simulink model "gtm_design"  (R2019b)
settings: Solver=ode3  StartTime=0.0  StopTime=Inf  FixedStep=Timestep  MaxStep=.1  RelTol=1e-5
InitFcn:
  | if ~exist('MAG3TempComp','var')
  |     appendmws(Cal_params_T2)
  | end
StopFcn:
  | MWSout=grabmws(bdroot);
  | MWSout.lastrun=datestr(now);
undefined symbols (not defined in the file): Aero, aftfuel, aftfuel_pos, b, bias, Cbar, cg_pos0, cg_shift_gear, DamageCase, DamageModels, DamageOnsetTime, engl_ang, engl_pos, engr_ang, engr_pos, fwdfuel, fwdfuel_pos, Inertia0, Inertia_shift_gear, ref_cg, runway_alt, S, StatesInp, symmetric_aero_on, Timestep, w0, WindDir, WindSpd
libraries: simulink_need_slupdate x28, Servo_Model_lib x18, simulink x4, Polyval_lib x3, GTM_aerolib x2, Cross_Product_3D_lib x2, Euler_to_DCM_lib x1, Vb_Converter_lib x1, eomlib x1, sensors_T2_design_lib x1, Doublet_Generator_lib x1, NamedStore_lib x1
(part 1 of 2)
settings Model: ExtModeAutoUpdateStatusClock=off  OrderedModelArguments=off  Creator=cox  LastModifiedBy=suvo
settings DataIOCC: LimitDataPoints=on  MaxDataPoints=50000  SaveFormat=Structure  SignalLoggingSaveFormat=ModelDataLogs  SaveOutput=off  SignalLogging=off  ReturnWorkspaceOutputs=off
settings OptimizationCC: BooleanDataType=off  ExpressionDepthLimit=2147483647  InitFltsAndDblsToZero=on  LifeSpan=inf
settings DebuggingCC: SaveWithParameterizedLinksMsg=none  UnderspecifiedInitializationDetection=Classic  MergeDetectMultiDrivingBlocksExec=none  SignalResolutionControl=TryResolveAllWithWarning  InheritedTsInSrcMsg=none  MultiTaskDSMMsg=warning  MultiTaskCondExecSysMsg=none  FcnCallInpInsideContextMsg=warning  StateNameClashWarn=warning  InitInArrayFormatMsg=none  SFUnexpectedBacktrackingDiag=warning  SFNoUnconditionalDefaultTransitionDiag=warning  SFExecutionAtInitializationDiag=none  ArithmeticOperatorsInVariantConditions=warning
settings HardwareCC: ProdBitPerPointer=32  ProdBitPerSizeT=32  ProdBitPerPtrDiffT=32  ProdLargestAtomicFloat=None  ProdIntDivRoundTo=Undefined  ProdEndianess=Unspecified  ProdWordSize=32  ProdHWDeviceType=32-bit Generic  TargetHWDeviceType=32-bit Generic
settings ModelReferenceCC: PropagateSignalLabelsOutOfModel=off
settings SFSimCC: SimUseLocalCustomCode=off  CustomCodeUndefinedFunction=UseInterfaceOnly
settings RTWCC: RTWUseLocalCustomCode=off
settings CodeAppCC: StateflowObjectComments=on
settings GRTTargetCC: TargetFcnLib=ansi_tfl_tmw.mat  TargetLangStandard=C89/C90 (ANSI)  CombineOutputUpdateFcns=off  GRTInterface=on
settings ConfigComp: CovMetricSettings=dw  CovHtmlReporting=on  CovSaveCumulativeToWorkspaceVar=on  CovSaveSingleToWorkspaceVar=on  CovExternalEMLEnable=off

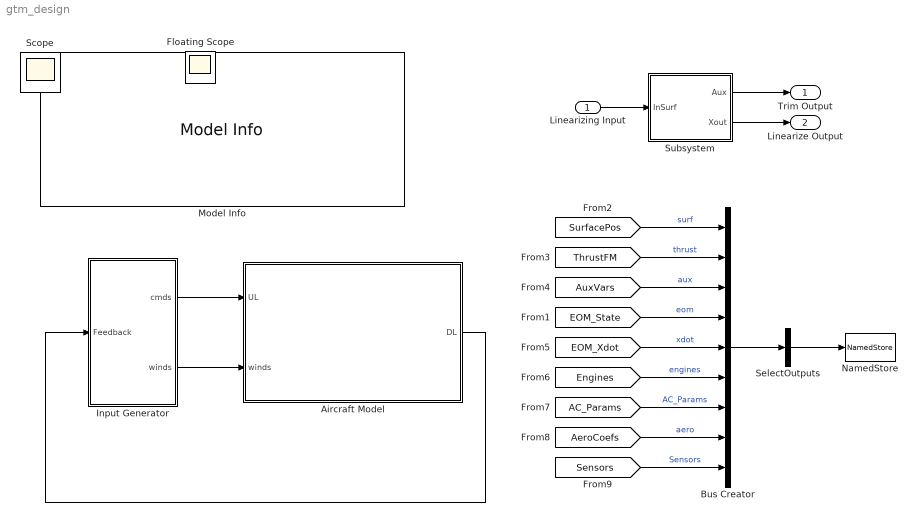
== system gtm_design ==
  Linearizing Input : Inport
  Aircraft Model : Subsystem  Tag=From trunk/GTMsim/gtm_model.mdl revision 162  BlockChoice=GTM_T2
      mask Display: image(imread('GTMtiny.png'))
  Bus Creator : BusCreator  Inputs=9
  Input Generator : Subsystem
  Model Info : simulink/Model-Wide Utilities/Model Info  Frame=on  DisplayStringWithTags=|  HorizontalTextAlignment=Center  LeftAlignmentValue=0.5
      | GTM Design-Simulation Model
      | Subversion Info: %<ModelVersion>
      | Last modified by %<LastModifiedBy> on %<LastModificationDate>
      | 
      | Copyright 2009
      | United States Government as represented by the 
      | Administrator of the National and Aeronautics and Space Administration.
      | 
      | No copyright is claimed in the United States under Title 17, U.S. Code.
      | All Other Rights Reserved.
  NamedStore : NamedStore_lib/NamedStore  Npts=inf  VarName=sout  expand=off
  SelectOutputs : BusSelector  OutputSignals=aux.eas,aux.alpha,aux.beta,aux.gamma  OutputAsBus=on
  Subsystem : Subsystem
  Trim Output : Outport  VectorParamsAs1DForOutWhenUnconnected=off
  Linearize Output : Outport  Port=2  VectorParamsAs1DForOutWhenUnconnected=off
  Floating Scope : Scope
  Scope : Scope
  wires:
  SelectOutputs/1 -> NamedStore/1
  [SurfacePos] -> Bus Creator/1  "surf"
  Linearizing Input/1 -> Subsystem/1(InSurf)
  Subsystem/1(Aux) -> Trim Output/1
  [EOM_State] -> Bus Creator/4  "eom"
  [AuxVars] -> Bus Creator/3  "aux"
  [ThrustFM] -> Bus Creator/2  "thrust"
  Subsystem/2(Xout) -> Linearize Output/1
  [EOM_Xdot] -> Bus Creator/5  "xdot"
  [Engines] -> Bus Creator/6  "engines"
  [AC_Params] -> Bus Creator/7  "AC_Params"
  Bus Creator/1 -> SelectOutputs/1
  Input Generator/1(cmds) -> Aircraft Model/1(UL)
  Input Generator/2(winds) -> Aircraft Model/2(winds)
  Aircraft Model/1(DL) -> Input Generator/1(Feedback)
  [AeroCoefs] -> Bus Creator/8  "aero"
  [Sensors] -> Bus Creator/9  "Sensors"

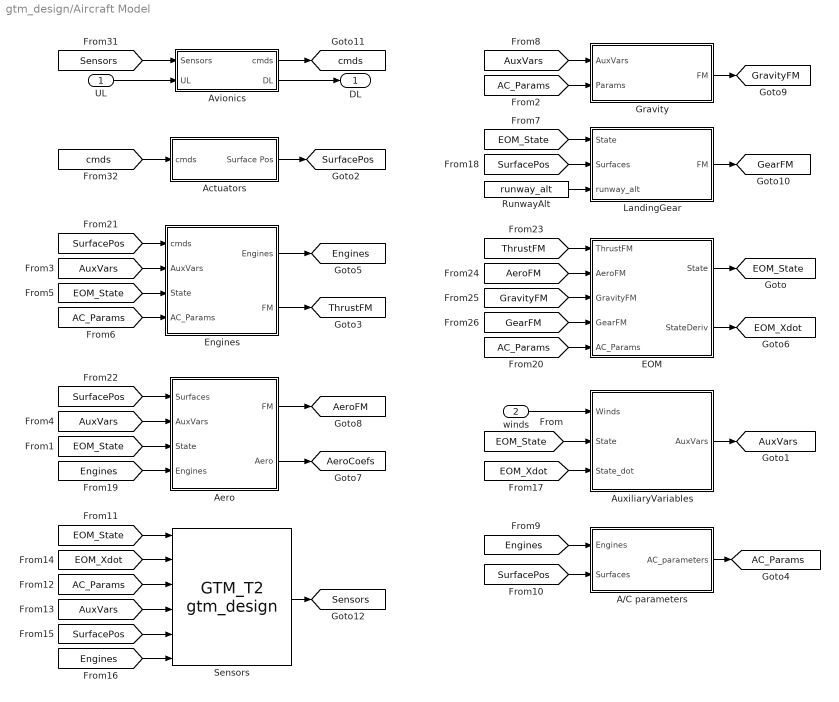
== system gtm_design/Aircraft Model ==
  UL : Inport
  winds : Inport  Port=2  PortDimensions=3
  A/C parameters : Subsystem
  Actuators : Subsystem
  Aero : Subsystem
  AuxiliaryVariables : Subsystem
  Avionics : Subsystem
  EOM : Subsystem
  Engines : Subsystem
  Gravity : Subsystem
  LandingGear : Subsystem  mask(LandingGear){GEAR_SPRING=25*12, zeta=0.4, NoseWheelRate=0.15}
      mask prompts: GEAR_SPRING "Gear Spring Constant (lbs/ft)"; zeta "Damping Factor"; NoseWheelRate "Nose Wheel Sensitivity"
      mask help: Landing Gear Model
  RunwayAlt : Constant  Value=runway_alt
  Sensors : sensors_T2_design_lib/GTM_T2 gtm_design  SystemSampleTime=-1  Latency=0  AutoFrameSizeCalculation=off
  DL : Outport  VectorParamsAs1DForOutWhenUnconnected=off
  tag scope: AC_Params=global, AeroCoefs=global, AeroFM=global, AuxVars=global, EOM_State=global, EOM_Xdot=global, Engines=global, GearFM=global, GravityFM=global, Sensors=global, SurfacePos=global, ThrustFM=global, cmds=global
  wires:
  Sensors/1 -> [Sensors]
  [cmds] -> Actuators/1(cmds)
  [Sensors] -> Avionics/1(Sensors)
  Avionics/1(cmds) -> [cmds]
  winds/1 -> AuxiliaryVariables/1(Winds)
  Actuators/1(Surface Pos) -> [SurfacePos]
  LandingGear/1(FM) -> [GearFM]
  [SurfacePos] -> LandingGear/2(Surfaces)
  [EOM_State] -> LandingGear/1(State)
  [EOM_State] -> Aero/3(State)
  AuxiliaryVariables/1(AuxVars) -> [AuxVars]
  [AuxVars] -> Aero/2(AuxVars)
  Aero/1(FM) -> [AeroFM]
  Engines/2(FM) -> [ThrustFM]
  EOM/1(State) -> [EOM_State]
  [AC_Params] -> Gravity/2(Params)
  [AuxVars] -> Gravity/1(AuxVars)
  [EOM_State] -> Engines/3(State)
  [AuxVars] -> Engines/2(AuxVars)
  [AC_Params] -> Engines/4(AC_Params)
  A/C parameters/1(AC_parameters) -> [AC_Params]
  [Engines] -> A/C parameters/1(Engines)
  [SurfacePos] -> A/C parameters/2(Surfaces)
  Engines/1(Engines) -> [Engines]
  [EOM_Xdot] -> AuxiliaryVariables/3(State_dot)
  [Engines] -> Aero/4(Engines)
  EOM/2(StateDeriv) -> [EOM_Xdot]
  [SurfacePos] -> Engines/1(cmds)
  RunwayAlt/1 -> LandingGear/3(runway_alt)
  [SurfacePos] -> Aero/1(Surfaces)
  Aero/2(Aero) -> [AeroCoefs]
  [EOM_State] -> AuxiliaryVariables/2(State)
  [ThrustFM] -> EOM/1(ThrustFM)
  [AeroFM] -> EOM/2(AeroFM)
  [GravityFM] -> EOM/3(GravityFM)
  [GearFM] -> EOM/4(GearFM)
  [AC_Params] -> EOM/5(AC_Params)
  [EOM_State] -> Sensors/1
  [AC_Params] -> Sensors/3
  [SurfacePos] -> Sensors/5
  [Engines] -> Sensors/6
  [EOM_Xdot] -> Sensors/2
  [AuxVars] -> Sensors/4
  Gravity/1(FM) -> [GravityFM]
  Avionics/2(DL) -> DL/1
  UL/1 -> Avionics/2(UL)

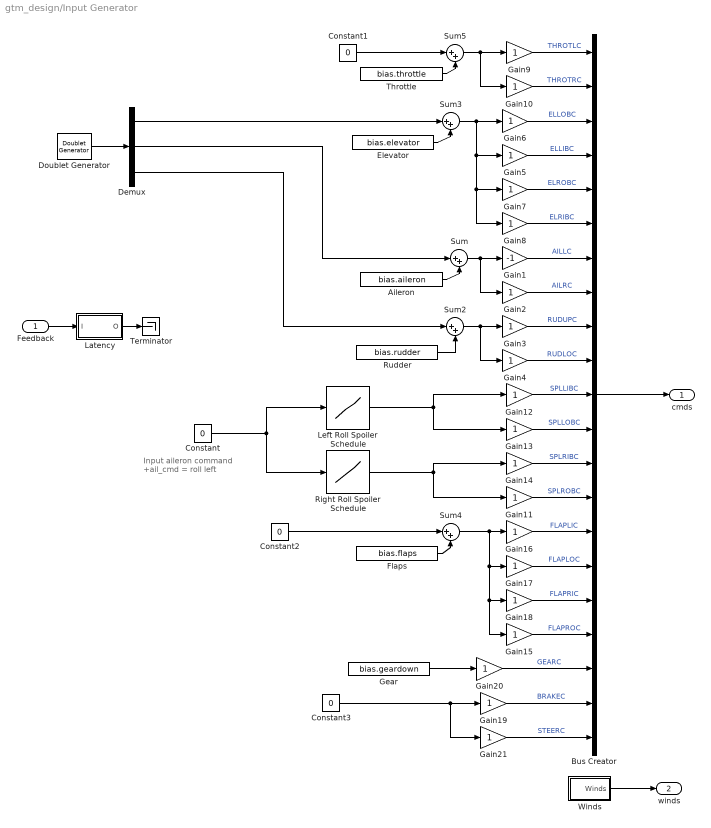
== system gtm_design/Input Generator ==
  note: Input aileron command
      | +ail_cmd = roll left
  Feedback : Inport
  Aileron : Constant  Value=bias.aileron
  Bus Creator : BusCreator  Inputs=21
  Constant{,1..3} (4 alike) : Constant  Value=0
  Demux : Demux  Outputs=3
  Doublet Generator : Doublet_Generator_lib/Doublet Generator  timeon=[2 12 7]  pulsewidth=[0.5 0.5 0.5]  amplitude=[0 0 0]
  Elevator : Constant  Value=bias.elevator
  Flaps : Constant  Value=bias.flaps
  Gain1 : Gain  Gain=-1  SaturateOnIntegerOverflow=on  OutDataTypeStr=Inherit: Same as input  ParamDataTypeStr=Inherit: Same as input
  Gain{2..21} (20 alike) : Gain  SaturateOnIntegerOverflow=on  OutDataTypeStr=Inherit: Same as input  ParamDataTypeStr=Inherit: Same as input
  Gear : Constant  Value=bias.geardown
  Latency : Subsystem
  Left Roll Spoiler Schedule : Lookup  InputValues="[-20\t-11.76\t-2.36\t0\t2.36\t11.76\t20\t]"  Table=[0 0 0 0 0 9 45]  LookUpMeth=Interpolation-Use End Values
  Right Roll Spoiler Schedule : Lookup  InputValues="[-20\t-11.76\t-2.36\t0\t2.36\t11.76\t20\t]"  Table=[45 9 0 0 0 0 0]  LookUpMeth=Interpolation-Use End Values
  Rudder : Constant  Value=bias.rudder
  Sum{,2..5} (5 alike) : Sum  Inputs=|++
  Terminator : Terminator
  Throttle : Constant  Value=bias.throttle
  Winds : Subsystem
  cmds : Outport  VectorParamsAs1DForOutWhenUnconnected=off
  winds : Outport  Port=2  VectorParamsAs1DForOutWhenUnconnected=off
  wires:
  Latency/1(O) -> Terminator/1
  Winds/1(Winds) -> winds/1
  Constant/1 -> Right Roll Spoiler Schedule/1, Left Roll Spoiler Schedule/1
  Right Roll Spoiler Schedule/1 -> Gain11/1, Gain14/1
  Left Roll Spoiler Schedule/1 -> Gain13/1, Gain12/1
  Gain12/1 -> Bus Creator/11  "SPLLIBC"
  Gain13/1 -> Bus Creator/12  "SPLLOBC"
  Gain14/1 -> Bus Creator/13  "SPLRIBC"
  Gain11/1 -> Bus Creator/14  "SPLROBC"
  Gain16/1 -> Bus Creator/15  "FLAPLIC"
  Gain17/1 -> Bus Creator/16  "FLAPLOC"
  Gain18/1 -> Bus Creator/17  "FLAPRIC"
  Gain15/1 -> Bus Creator/18  "FLAPROC"
  Gain9/1 -> Bus Creator/1  "THROTLC"
  Gain10/1 -> Bus Creator/2  "THROTRC"
  Gain5/1 -> Bus Creator/4  "ELLIBC"
  Gain6/1 -> Bus Creator/3  "ELLOBC"
  Gain7/1 -> Bus Creator/5  "ELROBC"
  Gain8/1 -> Bus Creator/6  "ELRIBC"
  Gain1/1 -> Bus Creator/7  "AILLC"
  Gain2/1 -> Bus Creator/8  "AILRC"
  Gain3/1 -> Bus Creator/9  "RUDUPC"
  Gain4/1 -> Bus Creator/10  "RUDLOC"
  Throttle/1 -> Sum5/2
  Constant1/1 -> Sum5/1
  Sum5/1 -> Gain10/1, Gain9/1
  Sum3/1 -> Gain6/1, Gain5/1, Gain7/1, Gain8/1
  Aileron/1 -> Sum/2
  Elevator/1 -> Sum3/2
  Sum/1 -> Gain1/1, Gain2/1
  Sum2/1 -> Gain3/1, Gain4/1
  Rudder/1 -> Sum2/2
  Flaps/1 -> Sum4/2
  Constant2/1 -> Sum4/1
  Sum4/1 -> Gain16/1, Gain17/1, Gain18/1, Gain15/1
  Doublet Generator/1 -> Demux/1
  Demux/2 -> Sum/1
  Demux/3 -> Sum2/1
  Gain19/1 -> Bus Creator/20  "BRAKEC"
  Gear/1 -> Gain20/1
  Constant3/1 -> Gain19/1, Gain21/1
  Demux/1 -> Sum3/1
  Bus Creator/1 -> cmds/1
  Feedback/1 -> Latency/1(I)
  Gain20/1 -> Bus Creator/19  "GEARC"
  Gain21/1 -> Bus Creator/21  "STEERC"

== system gtm_design/Subsystem ==
  InSurf : Inport
  Bus Selector : BusSelector  OutputSignals=eas,tas,alpha,beta,gamma,gndtrack  OutputAsBus=on
  Bus to Vector : BusToVector
  Bus to Vector1 : BusToVector
  DocBlock : simulink/Model-Wide Utilities/DocBlock  DocumentType=Text
      content=|
      | Inputs and Outputs selected here have a specific ordering.
      |
      |
      |
      | Do not change this without also changing output channel ordering in associated linmodel.m and
      | trimgtm.m functions
  Aux : Outport  VectorParamsAs1DForOutWhenUnconnected=off
  Xout : Outport  Port=2  VectorParamsAs1DForOutWhenUnconnected=off
  tag scope: SurfaceDeltas=global
  wires:
  [AuxVars] -> Bus Selector/1  "aux"
  [EOM_State] -> Bus to Vector1/1  "eom"
  Bus Selector/1 -> Bus to Vector/1
  InSurf/1 -> [SurfaceDeltas]
  Bus to Vector/1 -> Aux/1
  Bus to Vector1/1 -> Xout/1

== system gtm_design/Aircraft Model/A//C parameters ==
  Engines : Inport
  Surfaces : Inport  Port=2
  B : Constant  Value=b
  Bus Creator4 : BusCreator  Inputs=15
  Bus Selector : BusSelector  OutputSignals=fuel_used
  Bus Selector1 : BusSelector  OutputSignals=GEAR
  Cbar : Constant  Value=Cbar
  Demux : Demux  Outputs=6
  Inertia/Mass/CG Shift : Subsystem  mask{DamageModels=DamageModels}
      mask prompts: DamageModels "Array of Damage Cases"
      mask init:
      | Ncases=length(DamageModels);
      | dCGDamage=zeros(Ncases+1,3);   
      | dMassDamage=zeros(Ncases+1,1);
      | dInertiaDamage=zeros(Ncases+1,6);
      | for i=1:Ncases,
      |   if isfield(DamageModels{i},'Mass'),
      |      dInertiaDamage(i+1,:)=DamageModels{i}.Mass.dIxxIyyIzzIxzIyzIxy;
      |      dCGDamage(i+1,:)=DamageModels{i}.Mass.dCG;
      |      dMassDamage(i+1)=DamageModels{i}.Mass.dWeight;
      |   end
      | end
  S : Constant  Value=S
  TriggerDamage : Subsystem
  ixxb5 : Constant  Value=engr_pos
  ixxb6 : Constant  Value=engl_pos
  xCG1 : Constant  Value=ref_cg
  AC_parameters : Outport  VectorParamsAs1DForOutWhenUnconnected=off
  wires:
  Bus Selector/1 -> Inertia/Mass/CG Shift/2(fuel_used)  "<fuel_used>"
  Bus Selector1/1 -> Inertia/Mass/CG Shift/1(gear)  "<GEAR>"
  [DamageCase] -> Inertia/Mass/CG Shift/3(DamageCase)
  [DamageCase] -> Bus Creator4/13  "DamageCase"
  Inertia/Mass/CG Shift/3(CG) -> Bus Creator4/12  "CG"
  Inertia/Mass/CG Shift/2(mass) -> Bus Creator4/11  "mass"
  Demux/6 -> Bus Creator4/10  "Ixy"
  Demux/5 -> Bus Creator4/9  "Iyz"
  Demux/4 -> Bus Creator4/8  "Ixz"
  Demux/3 -> Bus Creator4/7  "Izz"
  Demux/2 -> Bus Creator4/6  "Iyy"
  Demux/1 -> Bus Creator4/5  "Ixx"
  ixxb6/1 -> Bus Creator4/15  "LfEng"
  ixxb5/1 -> Bus Creator4/14  "RtEng"
  xCG1/1 -> Bus Creator4/4  "CP"
  B/1 -> Bus Creator4/3  "B"
  Cbar/1 -> Bus Creator4/2  "Cbar"
  S/1 -> Bus Creator4/1  "S"
  TriggerDamage/1(damagecase) -> [DamageCase]
  Inertia/Mass/CG Shift/1(Inertia) -> Demux/1
  Surfaces/1 -> Bus Selector1/1
  Engines/1 -> Bus Selector/1
  Bus Creator4/1 -> AC_parameters/1

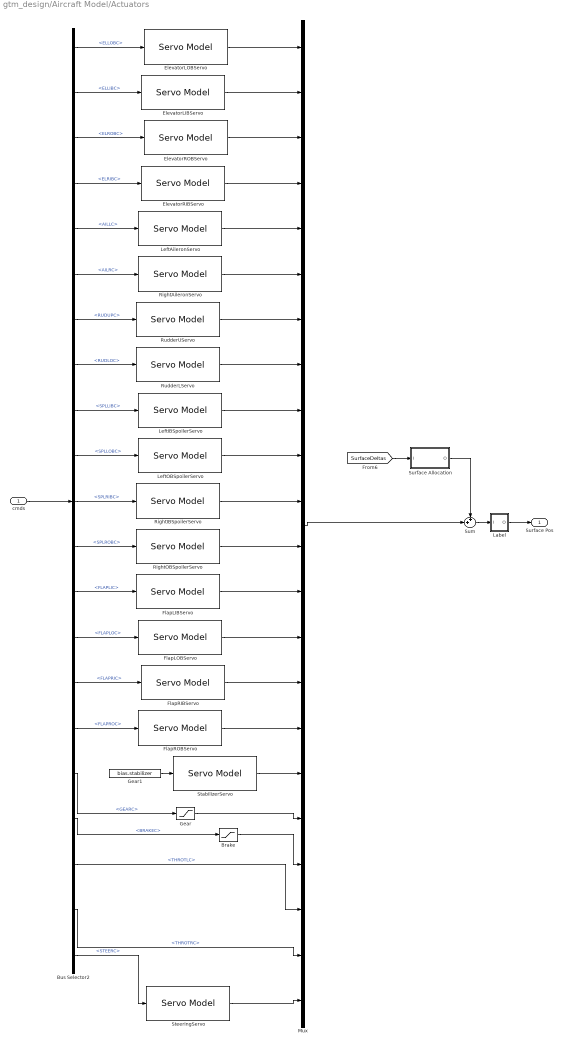
== system gtm_design/Aircraft Model/Actuators ==
  cmds : Inport
  Brake : Saturate  UpperLimit=1.0  LowerLimit=0.0
  Bus Selector2 : BusSelector  OutputSignals=ELLOBC,ELLIBC,ELROBC,ELRIBC,AILLC,AILRC,RUDUPC,RUDLOC,SPLLIBC,SPLLOBC,SPLRIBC,SPLROBC,FLAPLIC,FLAPLOC,FLAPRIC,FLAPROC,GEARC,BRAKEC,THROTLC,THROTRC,STEERC
  ElevatorLIBServo : Servo_Model_lib/Servo Model  freq=10  RL=300  POS_hi=20  POS_lo=-30  Bias=0
  ElevatorLOBServo : Servo_Model_lib/Servo Model  freq=10  RL=300  POS_hi=20  POS_lo=-30  Bias=0
  ElevatorRIBServo : Servo_Model_lib/Servo Model  freq=10  RL=300  POS_hi=20  POS_lo=-30  Bias=0
  ElevatorROBServo : Servo_Model_lib/Servo Model  freq=10  RL=300  POS_hi=20  POS_lo=-30  Bias=0
  FlapLIBServo : Servo_Model_lib/Servo Model  freq=10  RL=300  POS_hi=30  POS_lo=0  Bias=0
  FlapLOBServo : Servo_Model_lib/Servo Model  freq=10  RL=300  POS_hi=30  POS_lo=0  Bias=0
  FlapRIBServo : Servo_Model_lib/Servo Model  freq=10  RL=300  POS_hi=30  POS_lo=0  Bias=0
  FlapROBServo : Servo_Model_lib/Servo Model  freq=10  RL=300  POS_hi=30  POS_lo=0  Bias=0
  Gear : Saturate  UpperLimit=1.0  LowerLimit=0.0
  Gear1 : Constant  Value=bias.stabilizer
  Label : Subsystem
  LeftAileronServo : Servo_Model_lib/Servo Model  freq=10  RL=300  POS_hi=20.0  POS_lo=-20  Bias=0
  LeftIBSpoilerServo : Servo_Model_lib/Servo Model  freq=10  RL=300  POS_hi=15  POS_lo=0  Bias=0
  LeftOBSpoilerServo : Servo_Model_lib/Servo Model  freq=10  RL=300  POS_hi=45  POS_lo=0  Bias=0
  Mux : Mux  Inputs=22
  RightAileronServo : Servo_Model_lib/Servo Model  freq=10  RL=300  POS_hi=20.0  POS_lo=-20  Bias=0
  RightIBSpoilerServo : Servo_Model_lib/Servo Model  freq=10  RL=300  POS_hi=15  POS_lo=0  Bias=0
  RightOBSpoilerServo : Servo_Model_lib/Servo Model  freq=10  RL=300  POS_hi=45  POS_lo=0  Bias=0
  RudderLServo : Servo_Model_lib/Servo Model  freq=8.43  RL=300  POS_hi=30  POS_lo=-30.0  Bias=0
  RudderUServo : Servo_Model_lib/Servo Model  freq=8.43  RL=300  POS_hi=30  POS_lo=-30.0  Bias=0
  StabilizerServo : Servo_Model_lib/Servo Model  freq=10  RL=300  POS_hi=4  POS_lo=-12  Bias=0
  SteeringServo : Servo_Model_lib/Servo Model  freq=10  RL=300  POS_hi=30  POS_lo=0  Bias=0
  Sum : Sum  Inputs=++|
  Surface Allocation : Subsystem
  Surface Pos : Outport  VectorParamsAs1DForOutWhenUnconnected=off
  wires:
  SteeringServo/1 -> Mux/22
  Bus Selector2/21 -> SteeringServo/1  "<STEERC>"
  Bus Selector2/20 -> Mux/21  "<THROTRC>"
  Bus Selector2/19 -> Mux/20  "<THROTLC>"
  Gear1/1 -> StabilizerServo/1
  Surface Allocation/1(O) -> Sum/1
  cmds/1 -> Bus Selector2/1
  Brake/1 -> Mux/19
  Gear/1 -> Mux/18
  StabilizerServo/1 -> Mux/17
  FlapROBServo/1 -> Mux/16
  FlapRIBServo/1 -> Mux/15
  FlapLOBServo/1 -> Mux/14
  FlapLIBServo/1 -> Mux/13
  RightOBSpoilerServo/1 -> Mux/12
  RightIBSpoilerServo/1 -> Mux/11
  LeftOBSpoilerServo/1 -> Mux/10
  LeftIBSpoilerServo/1 -> Mux/9
  RudderLServo/1 -> Mux/8
  Bus Selector2/12 -> RightOBSpoilerServo/1  "<SPLROBC>"
  Bus Selector2/11 -> RightIBSpoilerServo/1  "<SPLRIBC>"
  Bus Selector2/10 -> LeftOBSpoilerServo/1  "<SPLLOBC>"
  Bus Selector2/9 -> LeftIBSpoilerServo/1  "<SPLLIBC>"
  Bus Selector2/8 -> RudderLServo/1  "<RUDLOC>"
  Bus Selector2/7 -> RudderUServo/1  "<RUDUPC>"
  RudderUServo/1 -> Mux/7
  RightAileronServo/1 -> Mux/6
  Bus Selector2/6 -> RightAileronServo/1  "<AILRC>"
  LeftAileronServo/1 -> Mux/5
  Bus Selector2/5 -> LeftAileronServo/1  "<AILLC>"
  ElevatorRIBServo/1 -> Mux/4
  Bus Selector2/4 -> ElevatorRIBServo/1  "<ELRIBC>"
  ElevatorROBServo/1 -> Mux/3
  Bus Selector2/3 -> ElevatorROBServo/1  "<ELROBC>"
  ElevatorLIBServo/1 -> Mux/2
  ElevatorLOBServo/1 -> Mux/1
  Bus Selector2/2 -> ElevatorLIBServo/1  "<ELLIBC>"
  Bus Selector2/1 -> ElevatorLOBServo/1  "<ELLOBC>"
  Mux/1 -> Sum/2
  Bus Selector2/18 -> Brake/1  "<BRAKEC>"
  Bus Selector2/17 -> Gear/1  "<GEARC>"
  Bus Selector2/16 -> FlapROBServo/1  "<FLAPROC>"
  Bus Selector2/15 -> FlapRIBServo/1  "<FLAPRIC>"
  Bus Selector2/14 -> FlapLOBServo/1  "<FLAPLOC>"
  Bus Selector2/13 -> FlapLIBServo/1  "<FLAPLIC>"
  [SurfaceDeltas] -> Surface Allocation/1(I)
  Label/1(O) -> Surface Pos/1
  Sum/1 -> Label/1(I)

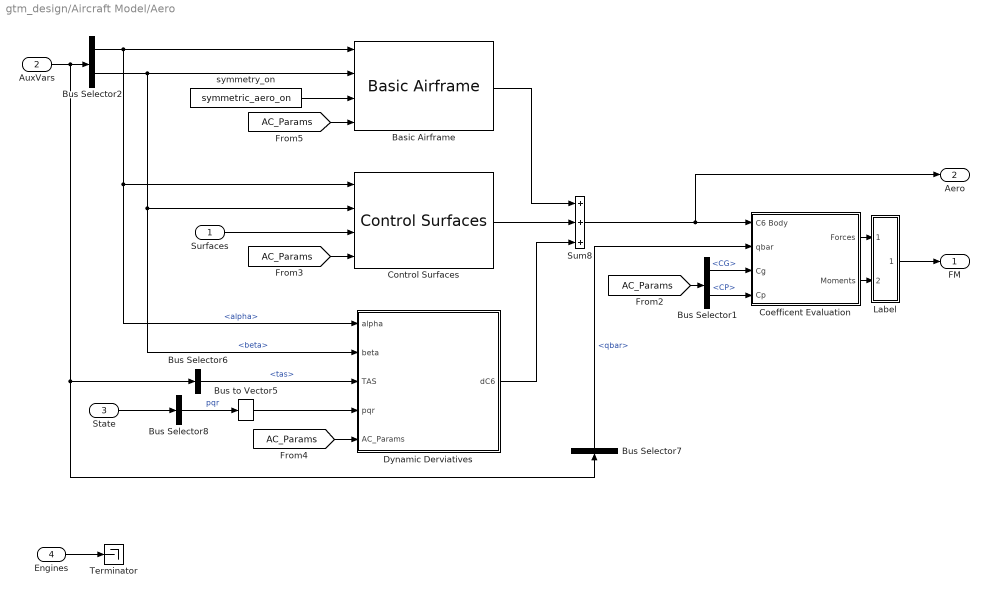
== system gtm_design/Aircraft Model/Aero ==
  Surfaces : Inport
  AuxVars : Inport  Port=2
  State : Inport  Port=3
  Engines : Inport  Port=4
  Basic Airframe : GTM_aerolib/Basic Airframe  SystemSampleTime=-1  Latency=0  AutoFrameSizeCalculation=off
  Bus Selector1 : BusSelector  OutputSignals=CG,CP
  Bus Selector2 : BusSelector  OutputSignals=alpha,beta
  Bus Selector6 : BusSelector  OutputSignals=tas
  Bus Selector7 : BusSelector  OutputSignals=qbar
  Bus Selector8 : BusSelector  OutputSignals=pb,qb,rb  OutputAsBus=on
  Bus to Vector5 : BusToVector
  Coefficent Evaluation : Subsystem  mask{b=b, cbar=Cbar, Sref=S}
      mask prompts: b "Reference Span (b)"; cbar "Reference Chord (cbar)"; Sref "Reference Area (Sref)"
      mask help:
      | Calulates the Force and Moments due to aerodynamic loads from vector of body axes aerodynamic coefficients:
      |    C6body = [Cx Cy Cz Cl Cm Cn].
      | Also requires dynamic pressure, cg/cp locations and reference lengths/area.
  Control Surfaces : GTM_aerolib/Control Surfaces  SystemSampleTime=-1  Latency=0  AutoFrameSizeCalculation=off
  Dynamic Derviatives : Subsystem  AncestorBlock=GTM_aerolib/Dynamic Derviatives
  Label : Subsystem
  Sum8 : Sum  Inputs=+++  SaturateOnIntegerOverflow=on  InputSameDT=on  OutDataTypeStr=Inherit: Same as first input
  Terminator : Terminator
  symmetry_on : Constant  Value=symmetric_aero_on
  FM : Outport  VectorParamsAs1DForOutWhenUnconnected=off
  Aero : Outport  Port=2  VectorParamsAs1DForOutWhenUnconnected=off
  wires:
  [AC_Params] -> Dynamic Derviatives/5(AC_Params)
  Bus to Vector5/1 -> Dynamic Derviatives/4(pqr)
  Bus Selector6/1 -> Dynamic Derviatives/3(TAS)  "<tas>"
  [AC_Params] -> Control Surfaces/4
  [AC_Params] -> Basic Airframe/4
  Bus Selector8/1 -> Bus to Vector5/1  "pqr"
  Engines/1 -> Terminator/1
  Basic Airframe/1 -> Sum8/1
  Control Surfaces/1 -> Sum8/2
  Dynamic Derviatives/1(dC6) -> Sum8/3
  State/1 -> Bus Selector8/1
  Bus Selector2/2 -> Basic Airframe/2, Dynamic Derviatives/2(beta), Control Surfaces/2  "<beta>"
  Bus Selector2/1 -> Basic Airframe/1, Dynamic Derviatives/1(alpha), Control Surfaces/1  "<alpha>"
  AuxVars/1 -> Bus Selector2/1, Bus Selector6/1, Bus Selector7/1
  Label/1(O) -> FM/1
  Bus Selector7/1 -> Coefficent Evaluation/2(qbar)  "<qbar>"
  Sum8/1 -> Aero/1, Coefficent Evaluation/1(C6 Body)
  Coefficent Evaluation/1(Forces) -> Label/1(If)
  Coefficent Evaluation/2(Moments) -> Label/2(Im)
  Bus Selector1/1 -> Coefficent Evaluation/3(Cg)  "<CG>"
  [AC_Params] -> Bus Selector1/1
  Bus Selector1/2 -> Coefficent Evaluation/4(Cp)  "<CP>"
  symmetry_on/1 -> Basic Airframe/3
  Surfaces/1 -> Control Surfaces/3

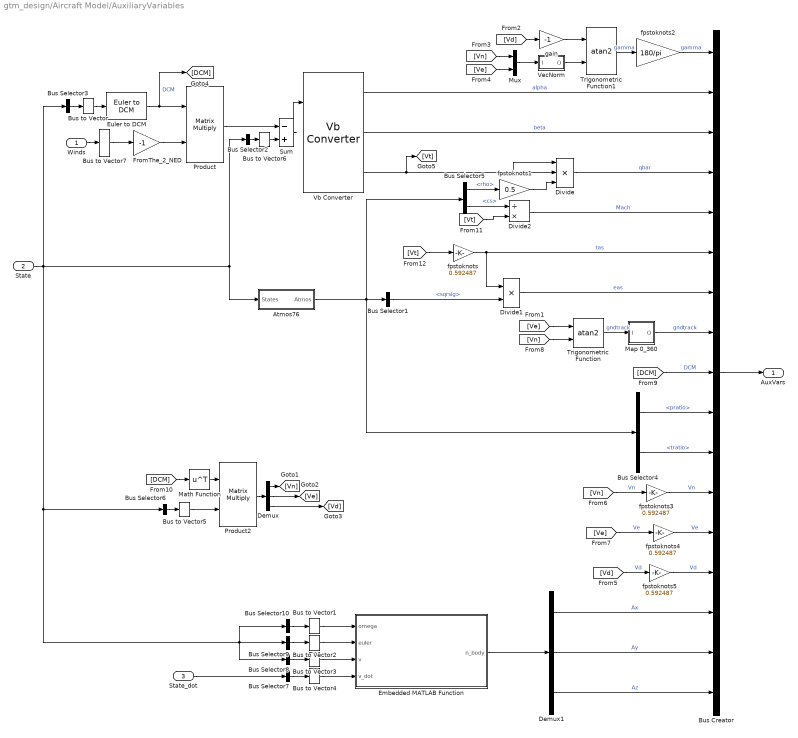
== system gtm_design/Aircraft Model/AuxiliaryVariables ==
  Winds : Inport  PortDimensions=3
  State : Inport  Port=2
  State_dot : Inport  Port=3
  Atmos76 : Subsystem
  Bus Creator : BusCreator  Inputs=17
  Bus Selector1 : BusSelector  OutputSignals=sqrsig
  Bus Selector10 : BusSelector  OutputSignals=pb,qb,rb  OutputAsBus=on
  Bus Selector2 : BusSelector  OutputSignals=ub,vb,wb  OutputAsBus=on
  Bus Selector3 : BusSelector  OutputSignals=phi,theta,psi  OutputAsBus=on
  Bus Selector4 : BusSelector  OutputSignals=pratio,tratio
  Bus Selector5 : BusSelector  OutputSignals=rho,cs
  Bus Selector6 : BusSelector  OutputSignals=ub,vb,wb  OutputAsBus=on
  Bus Selector7 : BusSelector  OutputSignals=ub_dot,vb_dot,wb_dot  OutputAsBus=on
  Bus Selector8 : BusSelector  OutputSignals=ub,vb,wb  OutputAsBus=on
  Bus Selector9 : BusSelector  OutputSignals=phi,theta,psi  OutputAsBus=on
  Bus to Vector{,1..7} (8 alike) : BusToVector
  Demux : Demux  Outputs=3
  Demux1 : Demux  Outputs=[1 1 1]
  Divide : Product  Inputs=***
  Divide1 : Product
  Divide2 : Product  Inputs=/*
  Embedded MATLAB Function : MATLAB Function  TreatAsAtomicUnit=on
  Euler to DCM : Euler_to_DCM_lib/Euler to DCM  SystemSampleTime=-1  Latency=0  AutoFrameSizeCalculation=off
  FromThe_2_NED : Gain  Gain=-1
  Map 0_360 : Subsystem
  Math Function : Math  Operator=transpose  SaturateOnIntegerOverflow=on
  Mux : Mux  Inputs=2
  Product : Product  Multiplication=Matrix(*)  RndMeth=Zero
  Product2 : Product  Multiplication=Matrix(*)  RndMeth=Zero
  Sum : Sum  Inputs=-+
  Trigonometric Function : Trigonometry  Operator=atan2
  Trigonometric Function1 : Trigonometry  Operator=atan2
  Vb Converter : Vb_Converter_lib/Vb Converter  SystemSampleTime=-1  Latency=0  AutoFrameSizeCalculation=off
  VecNorm : Subsystem
  fpstoknots{,3..5} (4 alike) : Gain  Gain=0.592487
  fpstoknots1 : Gain  Gain=0.5
  fpstoknots2 : Gain  Gain=180/pi
  gain : Gain  Gain=-1
  AuxVars : Outport  VectorParamsAs1DForOutWhenUnconnected=off
  wires:
  Bus to Vector7/1 -> FromThe_2_NED/1
  Bus to Vector6/1 -> Sum/2
  Bus Selector2/1 -> Bus to Vector6/1
  Bus to Vector5/1 -> Product2/2
  Bus to Vector4/1 -> Embedded MATLAB Function/4(v_dot)
  Bus to Vector3/1 -> Embedded MATLAB Function/3(v)
  Bus to Vector2/1 -> Embedded MATLAB Function/2(euler)
  Bus to Vector1/1 -> Embedded MATLAB Function/1(omega)
  Bus to Vector/1 -> Euler to DCM/1
  Bus Selector3/1 -> Bus to Vector/1
  Bus Selector6/1 -> Bus to Vector5/1
  [DCM] -> Math Function/1
  Product2/1 -> Demux/1
  Math Function/1 -> Product2/1
  Demux/1 -> [Vn]
  Demux/2 -> [Ve]
  Product/1 -> Sum/1
  Embedded MATLAB Function/1(n_body) -> Demux1/1
  Demux1/3 -> Bus Creator/17  "Az"
  Demux1/2 -> Bus Creator/16  "Ay"
  Demux1/1 -> Bus Creator/15  "Ax"
  Bus Selector10/1 -> Bus to Vector1/1
  Bus Selector9/1 -> Bus to Vector2/1
  Bus Selector8/1 -> Bus to Vector3/1
  State_dot/1 -> Bus Selector7/1
  Bus Selector7/1 -> Bus to Vector4/1
  Bus Creator/1 -> AuxVars/1
  [Vt] -> fpstoknots/1
  [Vt] -> Divide2/2
  [DCM] -> Bus Creator/9  "DCM"
  Sum/1 -> Vb Converter/1
  fpstoknots5/1 -> Bus Creator/14  "Vd"
  fpstoknots4/1 -> Bus Creator/13  "Ve"
  fpstoknots3/1 -> Bus Creator/12  "Vn"
  Divide2/1 -> Bus Creator/5  "Mach"
  Bus Selector5/2 -> Divide2/1  "<cs>"
  Trigonometric Function/1 -> Map 0_360/1(I)  "gndtrack"
  Map 0_360/1(O) -> Bus Creator/8  "gndtrack"
  [Vn] -> Trigonometric Function/2
  [Ve] -> Trigonometric Function/1
  Bus Selector4/2 -> Bus Creator/11  "<tratio>"
  Bus Selector4/1 -> Bus Creator/10  "<pratio>"
  [Vd] -> fpstoknots5/1  "Vd"
  [Vn] -> fpstoknots3/1  "Vn"
  [Ve] -> fpstoknots4/1  "Ve"
  FromThe_2_NED/1 -> Product/2
  Divide1/1 -> Bus Creator/7  "eas"
  State/1 -> Atmos76/1(States), Bus Selector2/1, Bus Selector6/1, Bus Selector8/1, Bus Selector10/1, Bus Selector9/1, Bus Selector3/1
  Atmos76/1(Atmos) -> Bus Selector4/1, Bus Selector1/1, Bus Selector5/1
  fpstoknots/1 -> Bus Creator/6, Divide1/1  "tas"
  Winds/1 -> Bus to Vector7/1
  Vb Converter/3 -> [Vt], Divide/1, Divide/2
  Bus Selector1/1 -> Divide1/2  "<sqrsig>"
  Vb Converter/1 -> Bus Creator/2  "alpha"
  Vb Converter/2 -> Bus Creator/3  "beta"
  Bus Selector5/1 -> fpstoknots1/1  "<rho>"
  fpstoknots1/1 -> Divide/3
  Divide/1 -> Bus Creator/4  "qbar"
  Euler to DCM/1 -> [DCM], Product/1  "DCM"
  Demux/3 -> [Vd]
  Trigonometric Function1/1 -> fpstoknots2/1  "gamma"
  gain/1 -> Trigonometric Function1/1
  [Vd] -> gain/1
  Mux/1 -> VecNorm/1(I)
  [Vn] -> Mux/1
  [Ve] -> Mux/2
  VecNorm/1(O) -> Trigonometric Function1/2
  fpstoknots2/1 -> Bus Creator/1  "gamma"

== system gtm_design/Aircraft Model/Avionics ==
  note: Downlink Path
  note: Uplink Path
  Sensors : Inport
  UL : Inport  Port=2
  cmds : Outport  VectorParamsAs1DForOutWhenUnconnected=off
  DL : Outport  Port=2  VectorParamsAs1DForOutWhenUnconnected=off
  wires:
  UL/1 -> cmds/1
  Sensors/1 -> DL/1

== system gtm_design/Aircraft Model/EOM ==
  ThrustFM : Inport
  AeroFM : Inport  Port=2
  GravityFM : Inport  Port=3
  GearFM : Inport  Port=4
  AC_Params : Inport  Port=5
  Add : Sum  Inputs=++++
  Aircraft 6DOF : eomlib/Aircraft 6DOF  UnitOfLength=ft
  Anti Windup : Subsystem
  Bus Selector1 : BusSelector  OutputSignals=Ixx,Iyy,Izz,Ixz,Iyz,Ixy  OutputAsBus=on
  Bus Selector11 : BusSelector  OutputSignals=mass
  Bus to Vector : BusToVector
  Bus to Vector1 : BusToVector
  Bus to Vector2 : BusToVector
  Constant : Constant  Value=[0 0 0]
  Integrator : Integrator  InitialCondition=StatesInp
  State Labels : Subsystem
  Xdot Labels : Subsystem
  State : Outport  VectorParamsAs1DForOutWhenUnconnected=off
  StateDeriv : Outport  Port=2  VectorParamsAs1DForOutWhenUnconnected=off
  wires:
  Bus to Vector2/1 -> Add/2
  Bus to Vector1/1 -> Add/1
  ThrustFM/1 -> Bus to Vector1/1
  AeroFM/1 -> Bus to Vector2/1
  State Labels/1(O) -> State/1
  Bus to Vector/1 -> Aircraft 6DOF/3
  GearFM/1 -> Add/4
  GravityFM/1 -> Add/3
  Add/1 -> Aircraft 6DOF/1
  Xdot Labels/1(O) -> StateDeriv/1
  Bus Selector1/1 -> Bus to Vector/1
  Aircraft 6DOF/1 -> Xdot Labels/1(I), Integrator/1
  Anti Windup/1(O) -> State Labels/1(I)
  Integrator/1 -> Aircraft 6DOF/5, Anti Windup/1(I)
  Bus Selector11/1 -> Aircraft 6DOF/2  "<mass>"
  AC_Params/1 -> Bus Selector1/1, Bus Selector11/1
  Constant/1 -> Aircraft 6DOF/4

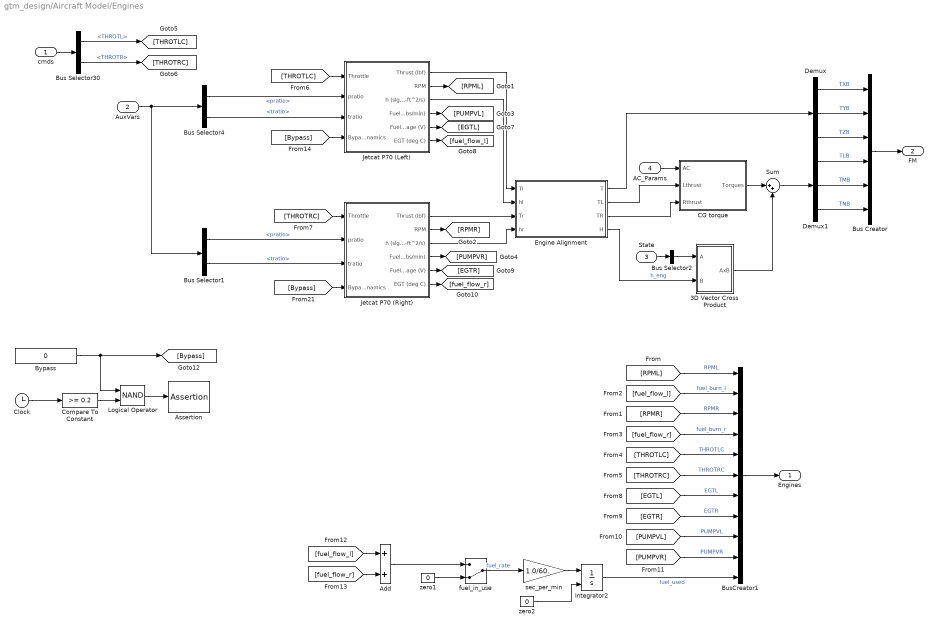
== system gtm_design/Aircraft Model/Engines ==
  cmds : Inport
  AuxVars : Inport  Port=2
  State : Inport  Port=3
  AC_Params : Inport  Port=4
  3D Vector Cross Product : Subsystem
  Add : Sum
  Assertion : Assertion  AssertionFailFcn=warndlg('Engine dynamics in bypass mode. Run setup.m to reset.','Warning!')
  Bus Creator : BusCreator  Inputs=6
  Bus Selector1 : BusSelector  OutputSignals=pratio,tratio
  Bus Selector2 : BusSelector  OutputSignals=pb,qb,rb  OutputAsBus=on
  Bus Selector30 : BusSelector  OutputSignals=THROTL,THROTR
  Bus Selector4 : BusSelector  OutputSignals=pratio,tratio
  BusCreator1 : BusCreator  Inputs=11
  Bypass : Constant  Value=0
  CG torque : Subsystem
  Clock : Clock
  Compare To Constant : simulink/Logic and Bit Operations/Compare To Constant  relop=>=  const=0.2  OutDataTypeStr=boolean  ZeroCross=off
  Demux : Demux  Outputs=3
  Demux1 : Demux  Outputs=3
  Engine Alignment : MATLAB Function  TreatAsAtomicUnit=on
  Integrator2 : Integrator  InitialConditionSource=external
  Jetcat P70 (Left) : Subsystem
      mask init:
      | % Curve fit parameters for Jetcat P70 Model
      | Coeff_thrust   = [0.000028864242464  -0.001914835880159 0.105916926095459  -1.251646340183624 ];
      | Coeff_throttle = [0.000033035538475  -0.008354385314499 1.191126728328792 31.518959847101669];
      | Coeff_fuelflow = [0.000046800927870  -0.000779344124807 0.122178501497750];
      | Coeff_tau      = [ -2.2400e-02   2.9948e+00];
      | Coeff_EGT      = [ 2E-5, -0.0036,0.2342,-8.0496,664.99]; %EGT model, deg C
      | fuelpump_table = [0 0.576	0.625	0.6985	0.7845	0.8575	0.919	0.9805	1.0415	1.1025...
      |                     1.1515	1.262	1.287	1.373	1.52	1.618	1.74	1.887	1.973...
      |                     2.12	2.255	2.4385	2.647	2.7575	2.9905	3.162]; %volts, table of fuel pump voltages
      | fuelflow_table = [0,0.0794,0.0876,0.102,0.1149,0.1275,0.1379,0.1487,0.1586,0.1671,...
      |                     0.1775,0.1858,0.194,0.2038,0.2206,0.2405,0.2566,0.2746,0.2921,0.3102,...
      |                     0.3266,0.3445,0.3533,0.3611,0.3866,0.4083;]*2; %lbs/min,   FULL fuel flow rates corresponding to pump voltages (fuelpump_table)  
      | % Equvalent Shaft parameters for engine
      | shaft_dia = 0.75/12.0;       % diameter of rotating turbine in feet 
      | shaft_len = 6.25/12.0;       % length of rotating turbine in feet   
      | density   = 15.2;            % mass density of steel in slugs/ft^3
  Jetcat P70 (Right) : Subsystem
      mask init: same as gtm_design/Aircraft Model/Engines/Jetcat P70 (Left)
  Logical Operator : Logic  Operator=NAND  AllPortsSameDT=off  OutDataTypeStr=boolean
  Sum : Sum  Inputs=|++
  fuel_in_use : ManualSwitch  CurrentSetting=0
  sec_per_min : Gain  Gain=1.0/60.  SaturateOnIntegerOverflow=on  OutDataTypeStr=Inherit: Same as input  ParamDataTypeStr=Inherit: Same as input
  zero1 : Constant  Value=0
  zero2 : Constant  Value=0
  Engines : Outport  VectorParamsAs1DForOutWhenUnconnected=off
  FM : Outport  Port=2  PortDimensions=6  VectorParamsAs1DForOutWhenUnconnected=off
  wires:
  Jetcat P70 (Right)/6(EGT (deg C)) -> [fuel_flow_r]
  Jetcat P70 (Right)/5(Fuel Pump Voltage (V)) -> [EGTR]
  Jetcat P70 (Left)/6(EGT (deg C)) -> [fuel_flow_l]
  Jetcat P70 (Left)/5(Fuel Pump Voltage (V)) -> [EGTL]
  cmds/1 -> Bus Selector30/1
  Demux/2 -> Bus Creator/2  "TYB"
  State/1 -> Bus Selector2/1
  Bus Selector2/1 -> 3D Vector Cross Product/1(A)
  Demux/3 -> Bus Creator/3  "TZB"
  Jetcat P70 (Left)/2(RPM) -> [RPML]
  Jetcat P70 (Left)/4(Fuel Flow (lbs/min)) -> [PUMPVL]
  Jetcat P70 (Right)/4(Fuel Flow (lbs/min)) -> [PUMPVR]
  Jetcat P70 (Right)/2(RPM) -> [RPMR]
  Bus Selector1/1 -> Jetcat P70 (Right)/2(pratio)  "<pratio>"
  Bus Selector1/2 -> Jetcat P70 (Right)/3(tratio)  "<tratio>"
  AuxVars/1 -> Bus Selector1/1, Bus Selector4/1
  AC_Params/1 -> CG torque/1(AC)
  Bus Creator/1 -> FM/1
  Bus Selector30/1 -> [THROTLC]  "<THROTL>"
  Bus Selector30/2 -> [THROTRC]  "<THROTR>"
  [THROTLC] -> Jetcat P70 (Left)/1(Throttle)
  [THROTRC] -> Jetcat P70 (Right)/1(Throttle)
  [THROTRC] -> BusCreator1/6  "THROTRC"
  [THROTLC] -> BusCreator1/5  "THROTLC"
  [fuel_flow_r] -> BusCreator1/4  "fuel_burn_r"
  [fuel_flow_l] -> BusCreator1/2  "fuel_burn_l"
  [RPMR] -> BusCreator1/3  "RPMR"
  [RPML] -> BusCreator1/1  "RPML"
  BusCreator1/1 -> Engines/1
  [EGTL] -> BusCreator1/7  "EGTL"
  [EGTR] -> BusCreator1/8  "EGTR"
  [PUMPVL] -> BusCreator1/9  "PUMPVL"
  [PUMPVR] -> BusCreator1/10  "PUMPVR"
  sec_per_min/1 -> Integrator2/1
  fuel_in_use/1 -> sec_per_min/1  "fuel_rate"
  Integrator2/1 -> BusCreator1/11  "fuel_used"
  zero2/1 -> Integrator2/2
  [fuel_flow_l] -> Add/1
  [fuel_flow_r] -> Add/2
  zero1/1 -> fuel_in_use/2
  Add/1 -> fuel_in_use/1
  Bus Selector4/1 -> Jetcat P70 (Left)/2(pratio)  "<pratio>"
  Bus Selector4/2 -> Jetcat P70 (Left)/3(tratio)  "<tratio>"
  [Bypass] -> Jetcat P70 (Left)/4(BypassDynamics)
  [Bypass] -> Jetcat P70 (Right)/4(BypassDynamics)
  Bypass/1 -> Logical Operator/1, [Bypass]
  Clock/1 -> Compare To Constant/1
  Jetcat P70 (Left)/1(Thrust (lbf)) -> Engine Alignment/1(Tl)
  Jetcat P70 (Right)/1(Thrust (lbf)) -> Engine Alignment/3(Tr)
  Demux/1 -> Bus Creator/1  "TXB"
  Jetcat P70 (Left)/3(h (slg-ft^2/s)) -> Engine Alignment/2(hl)
  Jetcat P70 (Right)/3(h (slg-ft^2/s)) -> Engine Alignment/4(hr)
  Engine Alignment/4(H) -> 3D Vector Cross Product/2(B)  "h_eng"
  Engine Alignment/1(T) -> Demux/1
  Engine Alignment/2(TL) -> CG torque/2(Lthrust)
  Engine Alignment/3(TR) -> CG torque/3(Rthrust)
  CG torque/1(Torques) -> Sum/1
  3D Vector Cross Product/1(AxB) -> Sum/2
  Sum/1 -> Demux1/1
  Demux1/1 -> Bus Creator/4  "TLB"
  Demux1/2 -> Bus Creator/5  "TMB"
  Demux1/3 -> Bus Creator/6  "TNB"
  Compare To Constant/1 -> Logical Operator/2
  Logical Operator/1 -> Assertion/1

== system gtm_design/Aircraft Model/Gravity ==
  AuxVars : Inport
  Params : Inport  Port=2
  Bus Selector1 : BusSelector  OutputSignals=DCM
  Bus Selector6 : BusSelector  OutputSignals=mass
  Ground : Ground
  Ground1 : Ground
  Mux : Mux  Inputs=[3 3]
  Mux1 : Mux  Inputs=3
  Product : Product  Multiplication=Matrix(*)  RndMeth=Zero
  Product1 : Product  RndMeth=Zero
  acc due to gravity : Constant  Value=32.17405
  FM : Outport  VectorParamsAs1DForOutWhenUnconnected=off
  wires:
  acc due to gravity/1 -> Product1/2
  Ground1/1 -> Mux/2
  Product1/1 -> Mux1/3
  Ground/1 -> Mux1/2, Mux1/1
  Mux1/1 -> Product/2
  Mux/1 -> FM/1
  Product/1 -> Mux/1
  Params/1 -> Bus Selector6/1
  AuxVars/1 -> Bus Selector1/1
  Bus Selector1/1 -> Product/1  "<DCM>"
  Bus Selector6/1 -> Product1/1  "<mass>"

== system gtm_design/Aircraft Model/LandingGear ==
  note: InAir
  State : Inport
  Surfaces : Inport  Port=2
  runway_alt : Inport  Port=3
  Bus Selector4 : BusSelector  OutputSignals=altitude
  Compare To Zero : simulink/Logic and Bit Operations/Compare To Zero  relop=<=  OutDataTypeStr=boolean  ZeroCross=off
  Constant : Constant  Value=zeros(6,1)
  LandingForces : Subsystem
  Logical Operator : Logic  Operator=NOT  AllPortsSameDT=off  OutDataTypeStr=boolean
  Sum : Sum  Inputs=-+|
  Switch : Switch  Criteria=u2 ~= 0  Threshold=.5
  FM : Outport  VectorParamsAs1DForOutWhenUnconnected=off
  wires:
  runway_alt/1 -> Sum/1
  State/1 -> Bus Selector4/1, LandingForces/2(Xeom)
  Bus Selector4/1 -> Sum/2  "<altitude>"
  Sum/1 -> Compare To Zero/1, LandingForces/1(h)
  Surfaces/1 -> LandingForces/3(Cmd)
  Compare To Zero/1 -> LandingForces/Enable, Logical Operator/1  "OnGround"
  Switch/1 -> FM/1
  LandingForces/1(Forces) -> Switch/3
  Constant/1 -> Switch/1
  Logical Operator/1 -> Switch/2

== system gtm_design/Input Generator/Latency ==
  I : Inport
  Unit Delay{,1..3} (4 alike) : UnitDelay  SampleTime=Timestep  HasFrameUpgradeWarning=on
  O : Outport  VectorParamsAs1DForOutWhenUnconnected=off
  wires:
  Unit Delay3/1 -> O/1
  Unit Delay2/1 -> Unit Delay3/1
  Unit Delay1/1 -> Unit Delay2/1
  Unit Delay/1 -> Unit Delay1/1
  I/1 -> Unit Delay/1

== system gtm_design/Input Generator/Winds ==
  Bus Creator3 : BusCreator  Inputs=3
  Ground9 : Ground
  Product1 : Product  Inputs=**  SaturateOnIntegerOverflow=on  InputSameDT=on  OutDataTypeStr=Inherit: Same as first input
  Product3 : Product  Inputs=**  SaturateOnIntegerOverflow=on  InputSameDT=on  OutDataTypeStr=Inherit: Same as first input
  Trigonometric Function : Trigonometry
  Trigonometric Function1 : Trigonometry  Operator=cos
  "WindDir (True, deg)" : Constant  Value=WindDir
  WindSpd (kts) : Constant  Value=WindSpd
  d2r : Gain  Gain=pi/180  SaturateOnIntegerOverflow=on  OutDataTypeStr=Inherit: Same as input  ParamDataTypeStr=Inherit: Same as input
  kts2fps : Gain  Gain=1.6889  SaturateOnIntegerOverflow=on  OutDataTypeStr=Inherit: Same as input  ParamDataTypeStr=Inherit: Same as input
  Winds : Outport  VectorParamsAs1DForOutWhenUnconnected=off
  wires:
  kts2fps/1 -> Product1/2, Product3/1
  WindSpd (kts)/1 -> kts2fps/1
  "WindDir (True, deg)"/1 -> d2r/1
  d2r/1 -> Trigonometric Function1/1, Trigonometric Function/1
  Trigonometric Function1/1 -> Product3/2
  Trigonometric Function/1 -> Product1/1
  Bus Creator3/1 -> Winds/1
  Ground9/1 -> Bus Creator3/3  "VerticalWind"
  Product1/1 -> Bus Creator3/2  "EastWind"
  Product3/1 -> Bus Creator3/1  "NorthWind"

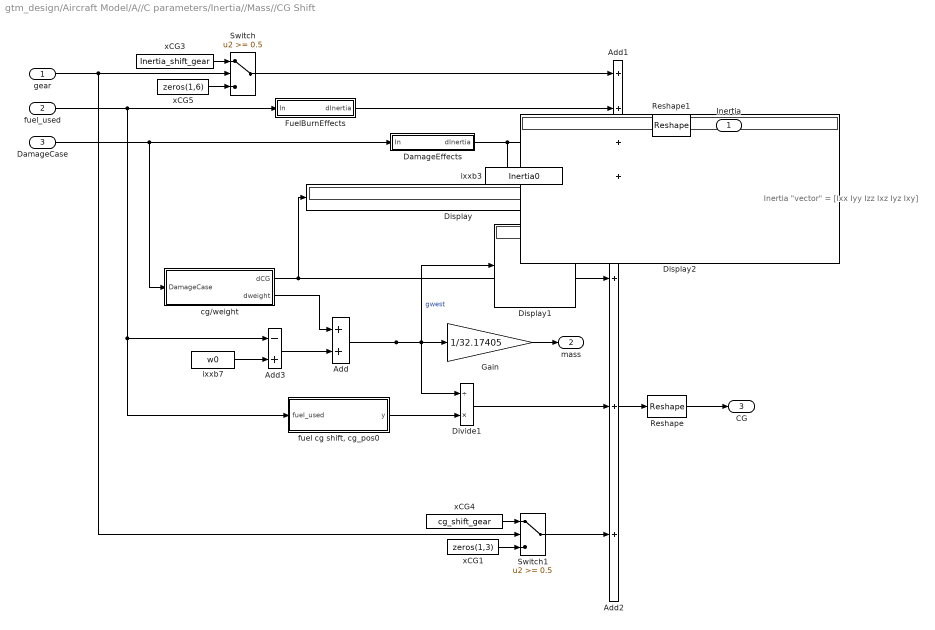
== system gtm_design/Aircraft Model/A//C parameters/Inertia//Mass//CG Shift ==
  note: Inertia "vector" = [Ixx Iyy Izz Ixz Iyz Ixy]
  gear : Inport
  fuel_used : Inport  Port=2
  DamageCase : Inport  Port=3
  Add : Sum
  Add1 : Sum  Inputs=++++
  Add2 : Sum  Inputs=+++
  Add3 : Sum  Inputs=-+
  DamageEffects : Subsystem
  Display : Display
  Display1 : Display
  Display2 : Display
  Divide1 : Product  Inputs=/*
  FuelBurnEffects : Subsystem
  Gain : Gain  Gain=1/32.17405
  Reshape : Reshape
  Reshape1 : Reshape
  Switch : Switch  Threshold=0.5
  Switch1 : Switch  Threshold=0.5
  cg/weight : Subsystem
  "fuel cg shift, cg_pos0" : MATLAB Function  TreatAsAtomicUnit=on
  ixxb3 : Constant  Value=Inertia0
  ixxb7 : Constant  Value=w0
  xCG1 : Constant  Value=zeros(1,3)
  xCG3 : Constant  Value=Inertia_shift_gear
  xCG4 : Constant  Value=cg_shift_gear
  xCG5 : Constant  Value=zeros(1,6)
  Inertia : Outport  VectorParamsAs1DForOutWhenUnconnected=off
  mass : Outport  Port=2  VectorParamsAs1DForOutWhenUnconnected=off
  CG : Outport  Port=3  VectorParamsAs1DForOutWhenUnconnected=off
  wires:
  "fuel cg shift, cg_pos0"/1(y) -> Divide1/2
  Divide1/1 -> Add2/2
  Reshape1/1 -> Inertia/1
  Reshape/1 -> CG/1
  cg/weight/2(dweight) -> Add/1
  gear/1 -> Switch1/2, Switch/2
  cg/weight/1(dCG) -> Display/1, Add2/1
  Add3/1 -> Add/2
  xCG1/1 -> Switch1/3
  xCG4/1 -> Switch1/1
  Switch1/1 -> Add2/3
  ixxb7/1 -> Add3/2
  Gain/1 -> mass/1
  Add2/1 -> Reshape/1
  Add/1 -> Display1/1, Divide1/1, Gain/1  "gwest"
  DamageCase/1 -> cg/weight/1(DamageCase), DamageEffects/1(In)
  DamageEffects/1(dInertia) -> Display2/1, Add1/3
  ixxb3/1 -> Add1/4
  fuel_used/1 -> "fuel cg shift, cg_pos0"/1(fuel_used), Add3/1, FuelBurnEffects/1(In)
  xCG5/1 -> Switch/3
  xCG3/1 -> Switch/1
  Add1/1 -> Reshape1/1
  Switch/1 -> Add1/1
  FuelBurnEffects/1(dInertia) -> Add1/2

== system gtm_design/Aircraft Model/A//C parameters/TriggerDamage ==
  Clock : Clock
  DamgeCase : Constant  Value=DamageCase
  Switch : Switch  Threshold=DamageOnsetTime
  Zero : Constant  Value=0
  damagecase : Outport  VectorParamsAs1DForOutWhenUnconnected=off
  wires:
  Clock/1 -> Switch/2
  Switch/1 -> damagecase/1
  Zero/1 -> Switch/3
  DamgeCase/1 -> Switch/1

== system gtm_design/Aircraft Model/Actuators/Label ==
  I : Inport
  Bus Creator : BusCreator  Inputs=22
  Demux : Demux  Outputs=22
  O : Outport  VectorParamsAs1DForOutWhenUnconnected=off
  wires:
  Demux/22 -> Bus Creator/22  "STEER"
  Demux/21 -> Bus Creator/21  "THROTR"
  Demux/20 -> Bus Creator/20  "THROTL"
  Demux/19 -> Bus Creator/19  "BRAKE"
  Demux/1 -> Bus Creator/1  "ELLOB"
  Demux/18 -> Bus Creator/18  "GEAR"
  Demux/17 -> Bus Creator/17  "STAB"
  Demux/16 -> Bus Creator/16  "FLAPROB"
  Demux/15 -> Bus Creator/15  "FLAPRIB"
  Demux/14 -> Bus Creator/14  "FLAPLOB"
  Demux/13 -> Bus Creator/13  "FLAPLIB"
  Demux/12 -> Bus Creator/12  "SPLROB"
  Demux/11 -> Bus Creator/11  "SPLRIB"
  Demux/10 -> Bus Creator/10  "SPLLOB"
  Demux/9 -> Bus Creator/9  "SPLLIB"
  Demux/8 -> Bus Creator/8  "RUDL"
  Demux/7 -> Bus Creator/7  "RUDU"
  Demux/6 -> Bus Creator/6  "AILR"
  Demux/5 -> Bus Creator/5  "AILL"
  Demux/4 -> Bus Creator/4  "ELRIB"
  Demux/3 -> Bus Creator/3  "ELROB"
  Demux/2 -> Bus Creator/2  "ELLIB"
  Bus Creator/1 -> O/1
  I/1 -> Demux/1

== system gtm_design/Aircraft Model/Actuators/Surface Allocation ==
  note: dStabilizer
  note: dthrottleL
  note: dthrottleR
  I : Inport
  Demux : Demux  Outputs=9
  Gain1 : Gain  Gain=-1
  Gain2 : Gain
  Ground1 : Ground
  Ground2 : Ground
  Ground5 : Ground
  Mux : Mux  Inputs=22
  O : Outport  VectorParamsAs1DForOutWhenUnconnected=off
  wires:
  Demux/7 -> Mux/17  "dStabilizer"
  Demux/6 -> Mux/16, Mux/15, Mux/13, Mux/14  "dFlap"
  Demux/5 -> Mux/12, Mux/11  "dR_Spo"
  Demux/4 -> Mux/10, Mux/9  "dL_Spo"
  Demux/1 -> Mux/4, Mux/3, Mux/2, Mux/1  "dElevator"
  Demux/2 -> Gain2/1, Gain1/1  "dAileron"
  Demux/9 -> Mux/21  "dthrottleR"
  Demux/8 -> Mux/20  "dthrottleL"
  Demux/3 -> Mux/8, Mux/7  "dRudder"
  Ground5/1 -> Mux/22  "dSteer"
  Ground2/1 -> Mux/19  "dbrake"
  Ground1/1 -> Mux/18  "dgear"
  Mux/1 -> O/1
  Gain2/1 -> Mux/6  "dR_Ail"
  Gain1/1 -> Mux/5  "dL_Ail"
  I/1 -> Demux/1

== system gtm_design/Aircraft Model/Aero/Coefficent Evaluation ==
  C6 Body : Inport
  qbar : Inport  Port=2
  Cg : Inport  Port=3
  Cp : Inport  Port=4
  3D Vector Cross Product : Subsystem
  Demux : Demux  Outputs=[3 3]
  Gain2 : Gain  Gain=Sref  SaturateOnIntegerOverflow=on  OutDataTypeStr=Inherit: Same as input  ParamDataTypeStr=Inherit: Same as input
  Product : Product  SaturateOnIntegerOverflow=on  InputSameDT=on  OutDataTypeStr=Inherit: Same as first input
  Reference Lengths : Gain  Gain=[b cbar b]  SaturateOnIntegerOverflow=on  OutDataTypeStr=Inherit: Same as input  ParamDataTypeStr=Inherit: Same as input
  Reshape : Reshape  OutputDimensionality=Column vector (2-D)  OutputDimensions=[3,1]
  Reshape1 : Reshape  OutputDimensions=[3,1]
  Sum : Sum  Inputs=-+  SaturateOnIntegerOverflow=on
  Sum1 : Sum  Inputs=++|  SaturateOnIntegerOverflow=on
  Forces : Outport  VectorParamsAs1DForOutWhenUnconnected=off
  Moments : Outport  Port=2  VectorParamsAs1DForOutWhenUnconnected=off
  wires:
  Sum/1 -> 3D Vector Cross Product/1(A)
  Cg/1 -> Sum/1
  Cp/1 -> Sum/2
  C6 Body/1 -> Product/1
  qbar/1 -> Product/2
  Product/1 -> Gain2/1
  Gain2/1 -> Demux/1
  Demux/2 -> Reference Lengths/1
  Demux/1 -> 3D Vector Cross Product/2(B), Forces/1
  Reference Lengths/1 -> Reshape/1
  Sum1/1 -> Reshape1/1
  3D Vector Cross Product/1(AxB) -> Sum1/1
  Reshape/1 -> Sum1/2
  Reshape1/1 -> Moments/1

== system gtm_design/Aircraft Model/Aero/Dynamic Derviatives ==
  alpha : Inport
  beta : Inport  Port=2
  TAS : Inport  Port=3
  pqr : Inport  Port=4
  AC_Params : Inport  Port=5
  AC_Params1 : InportShadow  Port=5
  AC_Params_Dup1 : InportShadow  Port=5
  Bus Selector : BusSelector  OutputSignals=DamageCase
  Data Type Conversion : DataTypeConversion  OutDataTypeStr=uint32  RndMeth=Nearest
  Forced Oscillation with Damage Increments : Subsystem
  Merge : Merge  InitialOutput=zeros(6,1)
  Rotary Blended UnDamaged Case : Subsystem
  Switch Case : SwitchCase  CaseConditions={[1,2,3,4,5,6]}
  TAS1 : InportShadow  Port=3
  alpha_Dup1 : InportShadow
  pqr_Dup1 : InportShadow  Port=4
  dC6 : Outport
  wires:
  Forced Oscillation with Damage Increments/1(dC6) -> Merge/1
  [ndx] -> Forced Oscillation with Damage Increments/5(DamageCase)
  AC_Params1/1 -> Forced Oscillation with Damage Increments/4(AC_Params)
  pqr_Dup1/1 -> Forced Oscillation with Damage Increments/3(pqr)
  TAS1/1 -> Forced Oscillation with Damage Increments/2(TAS)
  alpha_Dup1/1 -> Forced Oscillation with Damage Increments/1(alpha)
  [ndx] -> Switch Case/1
  Data Type Conversion/1 -> [ndx]
  AC_Params_Dup1/1 -> Bus Selector/1
  Bus Selector/1 -> Data Type Conversion/1  "<DamageCase>"
  Rotary Blended UnDamaged Case/1(dC6) -> Merge/2
  Switch Case/2 -> Rotary Blended UnDamaged Case/Action
  Switch Case/1 -> Forced Oscillation with Damage Increments/Action
  Merge/1 -> dC6/1
  AC_Params/1 -> Rotary Blended UnDamaged Case/5(AC_Params)
  pqr/1 -> Rotary Blended UnDamaged Case/4(pqr)
  TAS/1 -> Rotary Blended UnDamaged Case/3(TAS)
  beta/1 -> Rotary Blended UnDamaged Case/2(beta)
  alpha/1 -> Rotary Blended UnDamaged Case/1(alpha)

== system gtm_design/Aircraft Model/Aero/Label ==
  If : Inport
  Im : Inport  Port=2
  Bus Creator1 : BusCreator  Inputs=6
  Demux1 : Demux  Outputs=3
  Demux3 : Demux  Outputs=3
  O : Outport  VectorParamsAs1DForOutWhenUnconnected=off
  wires:
  Bus Creator1/1 -> O/1
  If/1 -> Demux1/1
  Demux1/1 -> Bus Creator1/1  "XB"
  Demux1/2 -> Bus Creator1/2  "YB"
  Demux1/3 -> Bus Creator1/3  "ZB"
  Demux3/1 -> Bus Creator1/4  "LB"
  Demux3/2 -> Bus Creator1/5  "MB"
  Demux3/3 -> Bus Creator1/6  "NB"
  Im/1 -> Demux3/1

== system gtm_design/Aircraft Model/AuxiliaryVariables/Atmos76 ==
  States : Inport
  Atmos List : Subsystem
  Bus Selector11 : BusSelector  OutputSignals=altitude
  Ground : Ground
  atmos76 : MATLAB Function  TreatAsAtomicUnit=on
  Atmos : Outport  VectorParamsAs1DForOutWhenUnconnected=off
  wires:
  Ground/1 -> atmos76/2(dt)
  Atmos List/1(O) -> Atmos/1
  States/1 -> Bus Selector11/1
  Bus Selector11/1 -> atmos76/1(z)  "<altitude>"
  atmos76/1(y) -> Atmos List/1(I)

== system gtm_design/Aircraft Model/AuxiliaryVariables/Map 0_360 ==
  I : Inport
  Constant : Constant  Value=2*pi
  Constant1 : Constant  Value=0
  Gain : Gain  Gain=180/pi
  Sum : Sum  Inputs=|++
  ifnegadd2pi : Switch
  O : Outport  VectorParamsAs1DForOutWhenUnconnected=off
  wires:
  Gain/1 -> O/1
  Constant1/1 -> ifnegadd2pi/1
  Constant/1 -> ifnegadd2pi/3
  ifnegadd2pi/1 -> Sum/2
  Sum/1 -> Gain/1
  I/1 -> ifnegadd2pi/2, Sum/1

== system gtm_design/Aircraft Model/AuxiliaryVariables/VecNorm ==
  I : Inport
  Math Function2 : Math  Operator=sqrt  SaturateOnIntegerOverflow=on
  Product : Product  RndMeth=Zero
  Sum of Elements : Sum  Inputs=+
  O : Outport  VectorParamsAs1DForOutWhenUnconnected=off
  wires:
  Math Function2/1 -> O/1
  I/1 -> Product/1, Product/2
  Product/1 -> Sum of Elements/1
  Sum of Elements/1 -> Math Function2/1

== system gtm_design/Aircraft Model/EOM/Anti Windup ==
  I : Inport
  Demux : Demux  Outputs=12
  Mux : Mux  Inputs=12
  Subsystem1 : Subsystem
      mask Display: disp('no windup 180')
  Subsystem3 : Subsystem
      mask Display: disp('no windup 180')
  Subsystem4 : Subsystem
      mask Display: disp('no windup 360')
  O : Outport  VectorParamsAs1DForOutWhenUnconnected=off
  wires:
  Mux/1 -> O/1
  Demux/11 -> Subsystem1/1(I)  "theta"
  Demux/10 -> Subsystem3/1(I)  "phi"
  Subsystem4/1(O) -> Mux/12  "psi"
  Subsystem1/1(O) -> Mux/11  "theta"
  Subsystem3/1(O) -> Mux/10  "phi"
  I/1 -> Demux/1
  Demux/1 -> Mux/1  "ub"
  Demux/2 -> Mux/2  "vb"
  Demux/3 -> Mux/3  "wb"
  Demux/4 -> Mux/4  "pb"
  Demux/5 -> Mux/5  "qb"
  Demux/6 -> Mux/6  "rb"
  Demux/7 -> Mux/7  "latitude"
  Demux/8 -> Mux/8  "longitude"
  Demux/9 -> Mux/9  "altitude"
  Demux/12 -> Subsystem4/1(I)  "psi"

== system gtm_design/Aircraft Model/EOM/State Labels ==
  I : Inport
  Bus Creator : BusCreator  Inputs=12
  Demux : Demux  Outputs=12
  O : Outport  VectorParamsAs1DForOutWhenUnconnected=off
  wires:
  Demux/12 -> Bus Creator/12  "psi"
  Demux/9 -> Bus Creator/9  "altitude"
  Demux/8 -> Bus Creator/8  "longitude"
  Demux/7 -> Bus Creator/7  "latitude"
  Demux/6 -> Bus Creator/6  "rb"
  Demux/5 -> Bus Creator/5  "qb"
  Demux/4 -> Bus Creator/4  "pb"
  Demux/3 -> Bus Creator/3  "wb"
  Demux/2 -> Bus Creator/2  "vb"
  Demux/1 -> Bus Creator/1  "ub"
  I/1 -> Demux/1
  Demux/10 -> Bus Creator/10  "phi"
  Demux/11 -> Bus Creator/11  "theta"
  Bus Creator/1 -> O/1

== system gtm_design/Aircraft Model/EOM/Xdot Labels ==
  I : Inport
  Bus Creator : BusCreator  Inputs=12
  Demux : Demux  Outputs=12
  O : Outport  VectorParamsAs1DForOutWhenUnconnected=off
  wires:
  Bus Creator/1 -> O/1
  Demux/11 -> Bus Creator/11  "theta_dot"
  Demux/10 -> Bus Creator/10  "phi_dot"
  I/1 -> Demux/1
  Demux/1 -> Bus Creator/1  "ub_dot"
  Demux/2 -> Bus Creator/2  "vb_dot"
  Demux/3 -> Bus Creator/3  "wb_dot"
  Demux/4 -> Bus Creator/4  "pb_dot"
  Demux/5 -> Bus Creator/5  "qb_dot"
  Demux/6 -> Bus Creator/6  "rb_dot"
  Demux/7 -> Bus Creator/7  "latitude_dot"
  Demux/8 -> Bus Creator/8  "longitude_dot"
  Demux/9 -> Bus Creator/9  "altitude_dot"
  Demux/12 -> Bus Creator/12  "psi_dot"

== system gtm_design/Aircraft Model/Engines/3D Vector Cross Product ==
  A : Inport
  B : Inport  Port=2
  Demux : Demux  Outputs=3
  Demux1 : Demux  Outputs=3
  Gain : Gain  Gain=-1  SaturateOnIntegerOverflow=on  OutDataTypeStr=Inherit: Same as input  ParamDataTypeStr=Inherit: Same as input
  Ground : Ground
  Mux : Mux  Inputs=9
  Product : Product  Multiplication=Matrix(*)  SaturateOnIntegerOverflow=on  OutDataTypeStr=Inherit: Same as first input
  Reshape : Reshape  OutputDimensionality=Customize  OutputDimensions=[3,3]
  AxB : Outport  VectorParamsAs1DForOutWhenUnconnected=off
  wires:
  B/1 -> Product/2
  Reshape/1 -> Product/1
  Mux/1 -> Reshape/1
  Demux1/1 -> Mux/8
  Demux/2 -> Mux/7
  Demux/1 -> Mux/6
  Demux1/3 -> Mux/4
  Demux1/2 -> Mux/3
  Demux/3 -> Mux/2
  Gain/1 -> Demux1/1
  Ground/1 -> Mux/9, Mux/5, Mux/1
  Product/1 -> AxB/1
  A/1 -> Gain/1, Demux/1

== system gtm_design/Aircraft Model/Engines/CG torque ==
  AC : Inport
  Lthrust : Inport  Port=2
  Rthrust : Inport  Port=3
  3D Vector Cross Product : Cross_Product_3D_lib/3D Vector Cross Product  SystemSampleTime=-1  Latency=0  AutoFrameSizeCalculation=off
  3D Vector Cross Product1 : Cross_Product_3D_lib/3D Vector Cross Product  SystemSampleTime=-1  Latency=0  AutoFrameSizeCalculation=off
  Bus Selector30 : BusSelector  OutputSignals=LfEng,CG,RtEng
  Sum1 : Sum  SaturateOnIntegerOverflow=on  InputSameDT=on  OutDataTypeStr=Inherit: Same as first input
  Sum6 : Sum  Inputs=+-  SaturateOnIntegerOverflow=on  InputSameDT=on  OutDataTypeStr=Inherit: Same as first input
  Sum7 : Sum  Inputs=-+  SaturateOnIntegerOverflow=on  InputSameDT=on  OutDataTypeStr=Inherit: Same as first input
  Torques : Outport  VectorParamsAs1DForOutWhenUnconnected=off
  wires:
  AC/1 -> Bus Selector30/1
  Bus Selector30/2 -> Sum7/1, Sum6/2  "<CG>"
  Lthrust/1 -> 3D Vector Cross Product1/2
  Rthrust/1 -> 3D Vector Cross Product/2
  Sum7/1 -> 3D Vector Cross Product/1
  Sum6/1 -> 3D Vector Cross Product1/1
  3D Vector Cross Product1/1 -> Sum1/1
  3D Vector Cross Product/1 -> Sum1/2
  Sum1/1 -> Torques/1
  Bus Selector30/3 -> Sum7/2  "<RtEng>"
  Bus Selector30/1 -> Sum6/1  "<LfEng>"
